simulink model "SVM_test2"  (R2020a)
settings: Solver=VariableStepAuto  StartTime=0.0  StopTime=Inf  FixedStep=Ts/2  RelTol=1e-3
PostLoadFcn:
  | , if any(exist('dsrtsu_mdlpostloadfcn', 'file') ~= 0), dsrtsu_mdlpostloadfcn('Execute', bdroot); end,
InitFcn:
  | , if any(exist('rtifpga_mdlclblib', 'file') ~= 0), rtifpga_mdlclblib('Init', bdroot); end,
model workspace (MAT data in the model file):
  FPGA_SVM_test2_1_Register_1_1_1_write : Simulink.Signal (value not decoded)
  FPGA_SVM_test2_1_Register_2_1_1_write : Simulink.Signal (value not decoded)
  FPGA_SVM_test2_1_Register_3_1_1_write : Simulink.Signal (value not decoded)
  FPGA_SVM_test2_1_Register_4_1_1_write : Simulink.Signal (value not decoded)
  FPGA_SVM_test2_1_Register_5_1_1_write : Simulink.Signal (value not decoded)
  FPGA_SVM_test2_1_Register_6_1_1_write : Simulink.Signal (value not decoded)
  FPGA_SVM_test2_1_Register_7_1_1_write : Simulink.Signal (value not decoded)
values from neighbouring files (symbols this model uses):
  clamp_threshold = 400    [param.m]
  i_fixed_gain = 10*1000/(3*100)    (= 33.3333333333)    [param.m]
  ioa_gain = 1    [param.m]
  ioa_offset = 0.09    [param.m]
  iob_gain = 1    [param.m]
  iob_offset = 0.06    [param.m]
  isa_gain = 1    [param.m]
  isa_offset = 0.1    [param.m]
  isb_gain = 1    [param.m]
  isb_offset = 0.3    [param.m]
  N = 1000    [param.m]
  vca_gain = 1    [param.m]
  vca_offset = 0.8    [param.m]
  vcb_gain = 1    [param.m]
  vcb_offset = 1.7    [param.m]
  vcc_gain = 1    [param.m]
  vcc_offset = 3    [param.m]
  vclamp_gain = 10*(76000+47000)/(3*100*2.5)    (= 1640)    [param.m]
  vclamp_offset = 11.7    [param.m]
  vi_fixed_gain = 10*33000/(3*100*2.5)    (= 440)    [param.m]
  via_gain = 1    [param.m]
  via_offset = 1    [param.m]
  vib_gain = 1    [param.m]
  vib_offset = 0.8    [param.m]
  vic_gain = 1    [param.m]
  vic_offset = -0.35    [param.m]
  voa_fixed_gain = 10*30000/(3*100*2.5)    (= 400)    [param.m]
  voa_gain = 1    [param.m]
  voa_offset = 0.7    [param.m]
libraries: xbsIndex_r4 x466, rti1202lib_adc_class1 x12, rtiproclib x10, simulink x3, rtifpgainterfacelib x1, powerlib_meascontrol x1
(part 8 of 9)

== system SVM_test2/Subsystem/FPGA_XDATA_READ_BL4 ==
  CEP1 : xbsIndex_r4/Clock Enable Probe  inherit_constraints=off  block_type=ceprobe
      settings: infoedit="Clock enable extractor.  Produces a Boolean output that mirrors the hardware clock enable associated with the input sample rate.<br><br>Hardware notes: in hardware this block costs nothing."
  CEP3 : xbsIndex_r4/Clock Enable Probe  inherit_constraints=off  block_type=ceprobe
      settings: infoedit="Clock enable extractor.  Produces a Boolean output that mirrors the hardware clock enable associated with the input sample rate.<br><br>Hardware notes: in hardware this block costs nothing."
  Constant1 : xbsIndex_r4/Constant  const=1  gui_display_data_type=Fixed-point  arith_type=Boolean  n_bits=16  bin_pt=14  preci_type=Single  exp_width=8  frac_width=24  explicit_period=on  period=1*1e-08  equ=P=C  opselect=C  inp2=PCIN>>17  opr=+  inp1=P  carry=CIN  dbl_ovrd=off  block_type=constant
  Constant3 : xbsIndex_r4/Constant  const=1  gui_display_data_type=Fixed-point  arith_type=Boolean  n_bits=16  bin_pt=14  preci_type=Single  exp_width=8  frac_width=24  explicit_period=on  period=1*1e-08  equ=P=C  opselect=C  inp2=PCIN>>17  opr=+  inp1=P  carry=CIN  dbl_ovrd=off  block_type=constant
  Delay1 : xbsIndex_r4/Delay  rst=off  infoeditControl=Selection of Reset will increase slice count due to use of real FFs and instead of SRLs  en=off  latency=0  reg_retiming=off  dbl_ovrd=off  block_type=delay
  Delay3 : xbsIndex_r4/Delay  rst=off  infoeditControl=Selection of Reset will increase slice count due to use of real FFs and instead of SRLs  en=off  latency=0  reg_retiming=off  dbl_ovrd=off  block_type=delay
  Register1 : xbsIndex_r4/Register  init=0  rst=off  en=on  dbl_ovrd=off  block_type=register
  Register3 : xbsIndex_r4/Register  init=0  rst=off  en=on  dbl_ovrd=off  block_type=register
  phs_read_register : Subsystem
      mask init: same as SVM_test2/Subsystem/FPGA_XDATA_READ_BL1/phs_read_register
  xreg_003_dout : xbsIndex_r4/Gateway In  gui_display_data_type=Fixed-point  arith_type=Unsigned  n_bits=32  bin_pt=0  preci_type=Single  exp_width=8  frac_width=24  rows=1  columns=1  quantization="Round  (unbiased: +/- Inf)"  overflow=Saturate  period=1e-08  UseAsADC=off  ADCChannel='1'  interface=None  automatic_assignment=on  address_offset=hex2dec('00')  intf_name=''  intf_description=''  default_value=0  timing_constraint=None  locs_specified=off  LOCs={}  io_standard={}  inherit_from_input=off  hdl_port=on  dbl_ovrd=off  block_type=gatewayin
  xreg_003_dout_wr : xbsIndex_r4/Gateway In  gui_display_data_type=Fixed-point  arith_type=Unsigned  n_bits=1  bin_pt=0  preci_type=Single  exp_width=8  frac_width=24  rows=1  columns=1  quantization="Round  (unbiased: +/- Inf)"  overflow=Saturate  period=1e-08  UseAsADC=off  ADCChannel='1'  interface=None  automatic_assignment=on  address_offset=hex2dec('00')  intf_name=''  intf_description=''  default_value=0  timing_constraint=None  locs_specified=off  LOCs={}  io_standard={}  inherit_from_input=off  hdl_port=on  dbl_ovrd=off  block_type=gatewayin
  Data : Outport
  Data New : Outport  Port=2
  wires:
  [FPGA_SVM_test2_rtiFPGAtmp_1_Register_4_1_1_write] -> phs_read_register/1(data_i)
  phs_read_register/2(data_new_o) -> xreg_003_dout_wr/1
  phs_read_register/1(data_o) -> xreg_003_dout/1
  xreg_003_dout_wr/1 -> Register3/1
  CEP3/1 -> Register3/2
  Constant3/1 -> CEP3/1
  Delay3/1 -> Data New/1
  Register3/1 -> Delay3/1
  xreg_003_dout/1 -> Register1/1
  CEP1/1 -> Register1/2
  Constant1/1 -> CEP1/1
  Delay1/1 -> Data/1
  Register1/1 -> Delay1/1

== system SVM_test2/Subsystem/FPGA_XDATA_READ_BL5 ==
  CEP1 : xbsIndex_r4/Clock Enable Probe  inherit_constraints=off  block_type=ceprobe
      settings: infoedit="Clock enable extractor.  Produces a Boolean output that mirrors the hardware clock enable associated with the input sample rate.<br><br>Hardware notes: in hardware this block costs nothing."
  CEP3 : xbsIndex_r4/Clock Enable Probe  inherit_constraints=off  block_type=ceprobe
      settings: infoedit="Clock enable extractor.  Produces a Boolean output that mirrors the hardware clock enable associated with the input sample rate.<br><br>Hardware notes: in hardware this block costs nothing."
  Constant1 : xbsIndex_r4/Constant  const=1  gui_display_data_type=Fixed-point  arith_type=Boolean  n_bits=16  bin_pt=14  preci_type=Single  exp_width=8  frac_width=24  explicit_period=on  period=1*1e-08  equ=P=C  opselect=C  inp2=PCIN>>17  opr=+  inp1=P  carry=CIN  dbl_ovrd=off  block_type=constant
  Constant3 : xbsIndex_r4/Constant  const=1  gui_display_data_type=Fixed-point  arith_type=Boolean  n_bits=16  bin_pt=14  preci_type=Single  exp_width=8  frac_width=24  explicit_period=on  period=1*1e-08  equ=P=C  opselect=C  inp2=PCIN>>17  opr=+  inp1=P  carry=CIN  dbl_ovrd=off  block_type=constant
  Delay1 : xbsIndex_r4/Delay  rst=off  infoeditControl=Selection of Reset will increase slice count due to use of real FFs and instead of SRLs  en=off  latency=0  reg_retiming=off  dbl_ovrd=off  block_type=delay
  Delay3 : xbsIndex_r4/Delay  rst=off  infoeditControl=Selection of Reset will increase slice count due to use of real FFs and instead of SRLs  en=off  latency=0  reg_retiming=off  dbl_ovrd=off  block_type=delay
  Register1 : xbsIndex_r4/Register  init=0  rst=off  en=on  dbl_ovrd=off  block_type=register
  Register3 : xbsIndex_r4/Register  init=0  rst=off  en=on  dbl_ovrd=off  block_type=register
  phs_read_register : Subsystem
      mask init: same as SVM_test2/Subsystem/FPGA_XDATA_READ_BL1/phs_read_register
  xreg_004_dout : xbsIndex_r4/Gateway In  gui_display_data_type=Fixed-point  arith_type=Unsigned  n_bits=32  bin_pt=0  preci_type=Single  exp_width=8  frac_width=24  rows=1  columns=1  quantization="Round  (unbiased: +/- Inf)"  overflow=Saturate  period=1e-08  UseAsADC=off  ADCChannel='1'  interface=None  automatic_assignment=on  address_offset=hex2dec('00')  intf_name=''  intf_description=''  default_value=0  timing_constraint=None  locs_specified=off  LOCs={}  io_standard={}  inherit_from_input=off  hdl_port=on  dbl_ovrd=off  block_type=gatewayin
  xreg_004_dout_wr : xbsIndex_r4/Gateway In  gui_display_data_type=Fixed-point  arith_type=Unsigned  n_bits=1  bin_pt=0  preci_type=Single  exp_width=8  frac_width=24  rows=1  columns=1  quantization="Round  (unbiased: +/- Inf)"  overflow=Saturate  period=1e-08  UseAsADC=off  ADCChannel='1'  interface=None  automatic_assignment=on  address_offset=hex2dec('00')  intf_name=''  intf_description=''  default_value=0  timing_constraint=None  locs_specified=off  LOCs={}  io_standard={}  inherit_from_input=off  hdl_port=on  dbl_ovrd=off  block_type=gatewayin
  Data : Outport
  Data New : Outport  Port=2
  wires:
  [FPGA_SVM_test2_rtiFPGAtmp_1_Register_5_1_1_write] -> phs_read_register/1(data_i)
  phs_read_register/2(data_new_o) -> xreg_004_dout_wr/1
  phs_read_register/1(data_o) -> xreg_004_dout/1
  xreg_004_dout_wr/1 -> Register3/1
  CEP3/1 -> Register3/2
  Constant3/1 -> CEP3/1
  Delay3/1 -> Data New/1
  Register3/1 -> Delay3/1
  xreg_004_dout/1 -> Register1/1
  CEP1/1 -> Register1/2
  Constant1/1 -> CEP1/1
  Delay1/1 -> Data/1
  Register1/1 -> Delay1/1

== system SVM_test2/Subsystem/FPGA_XDATA_READ_BL6 ==
  CEP1 : xbsIndex_r4/Clock Enable Probe  inherit_constraints=off  block_type=ceprobe
      settings: infoedit="Clock enable extractor.  Produces a Boolean output that mirrors the hardware clock enable associated with the input sample rate.<br><br>Hardware notes: in hardware this block costs nothing."
  CEP3 : xbsIndex_r4/Clock Enable Probe  inherit_constraints=off  block_type=ceprobe
      settings: infoedit="Clock enable extractor.  Produces a Boolean output that mirrors the hardware clock enable associated with the input sample rate.<br><br>Hardware notes: in hardware this block costs nothing."
  Constant1 : xbsIndex_r4/Constant  const=1  gui_display_data_type=Fixed-point  arith_type=Boolean  n_bits=16  bin_pt=14  preci_type=Single  exp_width=8  frac_width=24  explicit_period=on  period=1*1e-08  equ=P=C  opselect=C  inp2=PCIN>>17  opr=+  inp1=P  carry=CIN  dbl_ovrd=off  block_type=constant
  Constant3 : xbsIndex_r4/Constant  const=1  gui_display_data_type=Fixed-point  arith_type=Boolean  n_bits=16  bin_pt=14  preci_type=Single  exp_width=8  frac_width=24  explicit_period=on  period=1*1e-08  equ=P=C  opselect=C  inp2=PCIN>>17  opr=+  inp1=P  carry=CIN  dbl_ovrd=off  block_type=constant
  Delay1 : xbsIndex_r4/Delay  rst=off  infoeditControl=Selection of Reset will increase slice count due to use of real FFs and instead of SRLs  en=off  latency=0  reg_retiming=off  dbl_ovrd=off  block_type=delay
  Delay3 : xbsIndex_r4/Delay  rst=off  infoeditControl=Selection of Reset will increase slice count due to use of real FFs and instead of SRLs  en=off  latency=0  reg_retiming=off  dbl_ovrd=off  block_type=delay
  Register1 : xbsIndex_r4/Register  init=0  rst=off  en=on  dbl_ovrd=off  block_type=register
  Register3 : xbsIndex_r4/Register  init=0  rst=off  en=on  dbl_ovrd=off  block_type=register
  phs_read_register : Subsystem
      mask init: same as SVM_test2/Subsystem/FPGA_XDATA_READ_BL1/phs_read_register
  xreg_005_dout : xbsIndex_r4/Gateway In  gui_display_data_type=Fixed-point  arith_type=Unsigned  n_bits=32  bin_pt=0  preci_type=Single  exp_width=8  frac_width=24  rows=1  columns=1  quantization="Round  (unbiased: +/- Inf)"  overflow=Saturate  period=1e-08  UseAsADC=off  ADCChannel='1'  interface=None  automatic_assignment=on  address_offset=hex2dec('00')  intf_name=''  intf_description=''  default_value=0  timing_constraint=None  locs_specified=off  LOCs={}  io_standard={}  inherit_from_input=off  hdl_port=on  dbl_ovrd=off  block_type=gatewayin
  xreg_005_dout_wr : xbsIndex_r4/Gateway In  gui_display_data_type=Fixed-point  arith_type=Unsigned  n_bits=1  bin_pt=0  preci_type=Single  exp_width=8  frac_width=24  rows=1  columns=1  quantization="Round  (unbiased: +/- Inf)"  overflow=Saturate  period=1e-08  UseAsADC=off  ADCChannel='1'  interface=None  automatic_assignment=on  address_offset=hex2dec('00')  intf_name=''  intf_description=''  default_value=0  timing_constraint=None  locs_specified=off  LOCs={}  io_standard={}  inherit_from_input=off  hdl_port=on  dbl_ovrd=off  block_type=gatewayin
  Data : Outport
  Data New : Outport  Port=2
  wires:
  [FPGA_SVM_test2_rtiFPGAtmp_1_Register_6_1_1_write] -> phs_read_register/1(data_i)
  phs_read_register/2(data_new_o) -> xreg_005_dout_wr/1
  phs_read_register/1(data_o) -> xreg_005_dout/1
  xreg_005_dout_wr/1 -> Register3/1
  CEP3/1 -> Register3/2
  Constant3/1 -> CEP3/1
  Delay3/1 -> Data New/1
  Register3/1 -> Delay3/1
  xreg_005_dout/1 -> Register1/1
  CEP1/1 -> Register1/2
  Constant1/1 -> CEP1/1
  Delay1/1 -> Data/1
  Register1/1 -> Delay1/1

== system SVM_test2/Subsystem/FPGA_XDATA_READ_BL7 ==
  CEP1 : xbsIndex_r4/Clock Enable Probe  inherit_constraints=off  block_type=ceprobe
      settings: infoedit="Clock enable extractor.  Produces a Boolean output that mirrors the hardware clock enable associated with the input sample rate.<br><br>Hardware notes: in hardware this block costs nothing."
  CEP3 : xbsIndex_r4/Clock Enable Probe  inherit_constraints=off  block_type=ceprobe
      settings: infoedit="Clock enable extractor.  Produces a Boolean output that mirrors the hardware clock enable associated with the input sample rate.<br><br>Hardware notes: in hardware this block costs nothing."
  Constant1 : xbsIndex_r4/Constant  const=1  gui_display_data_type=Fixed-point  arith_type=Boolean  n_bits=16  bin_pt=14  preci_type=Single  exp_width=8  frac_width=24  explicit_period=on  period=1*1e-08  equ=P=C  opselect=C  inp2=PCIN>>17  opr=+  inp1=P  carry=CIN  dbl_ovrd=off  block_type=constant
  Constant3 : xbsIndex_r4/Constant  const=1  gui_display_data_type=Fixed-point  arith_type=Boolean  n_bits=16  bin_pt=14  preci_type=Single  exp_width=8  frac_width=24  explicit_period=on  period=1*1e-08  equ=P=C  opselect=C  inp2=PCIN>>17  opr=+  inp1=P  carry=CIN  dbl_ovrd=off  block_type=constant
  Delay1 : xbsIndex_r4/Delay  rst=off  infoeditControl=Selection of Reset will increase slice count due to use of real FFs and instead of SRLs  en=off  latency=0  reg_retiming=off  dbl_ovrd=off  block_type=delay
  Delay3 : xbsIndex_r4/Delay  rst=off  infoeditControl=Selection of Reset will increase slice count due to use of real FFs and instead of SRLs  en=off  latency=0  reg_retiming=off  dbl_ovrd=off  block_type=delay
  Register1 : xbsIndex_r4/Register  init=0  rst=off  en=on  dbl_ovrd=off  block_type=register
  Register3 : xbsIndex_r4/Register  init=0  rst=off  en=on  dbl_ovrd=off  block_type=register
  phs_read_register : Subsystem
      mask init: same as SVM_test2/Subsystem/FPGA_XDATA_READ_BL1/phs_read_register
  xreg_006_dout : xbsIndex_r4/Gateway In  gui_display_data_type=Fixed-point  arith_type=Unsigned  n_bits=32  bin_pt=0  preci_type=Single  exp_width=8  frac_width=24  rows=1  columns=1  quantization="Round  (unbiased: +/- Inf)"  overflow=Saturate  period=1e-08  UseAsADC=off  ADCChannel='1'  interface=None  automatic_assignment=on  address_offset=hex2dec('00')  intf_name=''  intf_description=''  default_value=0  timing_constraint=None  locs_specified=off  LOCs={}  io_standard={}  inherit_from_input=off  hdl_port=on  dbl_ovrd=off  block_type=gatewayin
  xreg_006_dout_wr : xbsIndex_r4/Gateway In  gui_display_data_type=Fixed-point  arith_type=Unsigned  n_bits=1  bin_pt=0  preci_type=Single  exp_width=8  frac_width=24  rows=1  columns=1  quantization="Round  (unbiased: +/- Inf)"  overflow=Saturate  period=1e-08  UseAsADC=off  ADCChannel='1'  interface=None  automatic_assignment=on  address_offset=hex2dec('00')  intf_name=''  intf_description=''  default_value=0  timing_constraint=None  locs_specified=off  LOCs={}  io_standard={}  inherit_from_input=off  hdl_port=on  dbl_ovrd=off  block_type=gatewayin
  Data : Outport
  Data New : Outport  Port=2
  wires:
  [FPGA_SVM_test2_rtiFPGAtmp_1_Register_7_1_1_write] -> phs_read_register/1(data_i)
  phs_read_register/2(data_new_o) -> xreg_006_dout_wr/1
  phs_read_register/1(data_o) -> xreg_006_dout/1
  xreg_006_dout_wr/1 -> Register3/1
  CEP3/1 -> Register3/2
  Constant3/1 -> CEP3/1
  Delay3/1 -> Data New/1
  Register3/1 -> Delay3/1
  xreg_006_dout/1 -> Register1/1
  CEP1/1 -> Register1/2
  Constant1/1 -> CEP1/1
  Delay1/1 -> Data/1
  Register1/1 -> Delay1/1

== system SVM_test2/RTI Data/RTI Data Store/RTI Data Store ==
  RTI Data Store : Subsystem  mask(RTI_DATA_STORE){}
      mask help:
      | RTI Data Store Block. This block is used by RTI to store internal model dependent data. Deleting this block will result in data loss.
      |
      | NEVER DELETE, COPY, OR MODIFY THIS BLOCK!
      mask Help:
      | RTI Data Store Block. This block is used by RTI to store internal model dependent data. Deleting this block will result in data loss.
      | 
      | NEVER DELETE, COPY, OR MODIFY THIS BLOCK!
      mask Display: text(0.5, 0.5, ' ', 'HorizontalAlignment', 'center');

== system SVM_test2/Subsystem/FPGA_INT_BL1/phs_interrupt ==
  note: Subsystem simulating the communication
      | function specific behaviour. This is how the
      | FPGA framework driver takes effect on the data.
  note: Subsystem simulating the phs bus
      | access via RTLib functions.
  data_i : Inport
  com_fct_model : Subsystem
  phs/rtlib_sim_model : Subsystem
  data_o : Outport  VectorParamsAs1DForOutWhenUnconnected=off
  wires:
  data_i/1 -> com_fct_model/1(data_i1)
  com_fct_model/1(data_o1) -> phs/rtlib_sim_model/1(data_i1)
  phs/rtlib_sim_model/1(data_o1) -> data_o/1

== system SVM_test2/Subsystem/FPGA_INT_BL2/phs_interrupt ==
  note: Subsystem simulating the communication
      | function specific behaviour. This is how the
      | FPGA framework driver takes effect on the data.
  note: Subsystem simulating the phs bus
      | access via RTLib functions.
  data_i : Inport
  com_fct_model : Subsystem
  phs/rtlib_sim_model : Subsystem
  data_o : Outport  VectorParamsAs1DForOutWhenUnconnected=off
  wires:
  data_i/1 -> com_fct_model/1(data_i1)
  com_fct_model/1(data_o1) -> phs/rtlib_sim_model/1(data_i1)
  phs/rtlib_sim_model/1(data_o1) -> data_o/1

== system SVM_test2/Subsystem/FPGA_IO_WRITE_BL1/dig_inout_tp1 ==
  note: The Digital In value is simulated by Threshold voltage detection.
  note: The nominal input range is NOT simulated because
      | the HW does not saturate according to the input range.
  data_in_i : Inport
  enable_i : Inport  Port=2
  data_out_i : Inport  Port=3
  direction_i : Inport  Port=4
  Data Type Conversion : DataTypeConversion
  Data Type Conversion1 : DataTypeConversion
  Disabled Input Value : Constant  Value=0
  Disabled Output Value : Constant  Value=0
  Invert : Constant  Value=inverted_dio
  Invert1 : Constant  Value=inverted_dio
  Inverter : Logic  Operator=NOT  AllPortsSameDT=off  OutDataTypeStr=boolean
  Inverter1 : Logic  AllPortsSameDT=off  OutDataTypeStr=boolean
  Inverter2 : Logic  Operator=NOT  AllPortsSameDT=off  OutDataTypeStr=boolean
  Inverter3 : Logic  AllPortsSameDT=off  OutDataTypeStr=boolean
  Inverter4 : Logic  Operator=NOT  AllPortsSameDT=off  OutDataTypeStr=boolean
  Relational Operator : RelationalOperator  OutDataTypeStr=boolean  RndMeth=Nearest
  Switch{,1..3} (4 alike) : Switch  Threshold=1
  Threshold Voltage : Constant  Value=2
  Voltage : Gain  Gain=voltage  ParamDataTypeStr=float('double')
  data_in_o : Outport  VectorParamsAs1DForOutWhenUnconnected=off
  data_out_o : Outport  Port=2  VectorParamsAs1DForOutWhenUnconnected=off
  wires:
  data_in_i/1 -> Relational Operator/1
  Threshold Voltage/1 -> Relational Operator/2
  Disabled Input Value/1 -> Switch/3
  Switch1/1 -> data_in_o/1
  Invert/1 -> Switch1/2
  Inverter/1 -> Switch1/1
  Relational Operator/1 -> Switch/1
  Switch/1 -> Inverter/1, Switch1/3
  enable_i/1 -> Data Type Conversion/1
  Inverter1/1 -> Switch/2
  direction_i/1 -> Data Type Conversion1/1
  Inverter2/1 -> Inverter1/2
  Disabled Output Value/1 -> Switch2/3
  Inverter3/1 -> Switch2/2
  data_out_i/1 -> Switch2/1
  Invert1/1 -> Switch3/2
  Inverter4/1 -> Switch3/1
  Switch2/1 -> Inverter4/1, Switch3/3
  Switch3/1 -> Voltage/1
  Data Type Conversion/1 -> Inverter1/1, Inverter3/1
  Data Type Conversion1/1 -> Inverter2/1, Inverter3/2
  Voltage/1 -> data_out_o/1

== system SVM_test2/Subsystem/FPGA_IO_WRITE_BL10/dig_inout_tp1 ==
  note: The Digital In value is simulated by Threshold voltage detection.
  note: The nominal input range is NOT simulated because
      | the HW does not saturate according to the input range.
  data_in_i : Inport
  enable_i : Inport  Port=2
  data_out_i : Inport  Port=3
  direction_i : Inport  Port=4
  Data Type Conversion : DataTypeConversion
  Data Type Conversion1 : DataTypeConversion
  Disabled Input Value : Constant  Value=0
  Disabled Output Value : Constant  Value=0
  Invert : Constant  Value=inverted_dio
  Invert1 : Constant  Value=inverted_dio
  Inverter : Logic  Operator=NOT  AllPortsSameDT=off  OutDataTypeStr=boolean
  Inverter1 : Logic  AllPortsSameDT=off  OutDataTypeStr=boolean
  Inverter2 : Logic  Operator=NOT  AllPortsSameDT=off  OutDataTypeStr=boolean
  Inverter3 : Logic  AllPortsSameDT=off  OutDataTypeStr=boolean
  Inverter4 : Logic  Operator=NOT  AllPortsSameDT=off  OutDataTypeStr=boolean
  Relational Operator : RelationalOperator  OutDataTypeStr=boolean  RndMeth=Nearest
  Switch{,1..3} (4 alike) : Switch  Threshold=1
  Threshold Voltage : Constant  Value=2
  Voltage : Gain  Gain=voltage  ParamDataTypeStr=float('double')
  data_in_o : Outport  VectorParamsAs1DForOutWhenUnconnected=off
  data_out_o : Outport  Port=2  VectorParamsAs1DForOutWhenUnconnected=off
  wires:
  data_in_i/1 -> Relational Operator/1
  Threshold Voltage/1 -> Relational Operator/2
  Disabled Input Value/1 -> Switch/3
  Switch1/1 -> data_in_o/1
  Invert/1 -> Switch1/2
  Inverter/1 -> Switch1/1
  Relational Operator/1 -> Switch/1
  Switch/1 -> Inverter/1, Switch1/3
  enable_i/1 -> Data Type Conversion/1
  Inverter1/1 -> Switch/2
  direction_i/1 -> Data Type Conversion1/1
  Inverter2/1 -> Inverter1/2
  Disabled Output Value/1 -> Switch2/3
  Inverter3/1 -> Switch2/2
  data_out_i/1 -> Switch2/1
  Invert1/1 -> Switch3/2
  Inverter4/1 -> Switch3/1
  Switch2/1 -> Inverter4/1, Switch3/3
  Switch3/1 -> Voltage/1
  Data Type Conversion/1 -> Inverter1/1, Inverter3/1
  Data Type Conversion1/1 -> Inverter2/1, Inverter3/2
  Voltage/1 -> data_out_o/1

== system SVM_test2/Subsystem/FPGA_IO_WRITE_BL11/dig_inout_tp1 ==
  note: The Digital In value is simulated by Threshold voltage detection.
  note: The nominal input range is NOT simulated because
      | the HW does not saturate according to the input range.
  data_in_i : Inport
  enable_i : Inport  Port=2
  data_out_i : Inport  Port=3
  direction_i : Inport  Port=4
  Data Type Conversion : DataTypeConversion
  Data Type Conversion1 : DataTypeConversion
  Disabled Input Value : Constant  Value=0
  Disabled Output Value : Constant  Value=0
  Invert : Constant  Value=inverted_dio
  Invert1 : Constant  Value=inverted_dio
  Inverter : Logic  Operator=NOT  AllPortsSameDT=off  OutDataTypeStr=boolean
  Inverter1 : Logic  AllPortsSameDT=off  OutDataTypeStr=boolean
  Inverter2 : Logic  Operator=NOT  AllPortsSameDT=off  OutDataTypeStr=boolean
  Inverter3 : Logic  AllPortsSameDT=off  OutDataTypeStr=boolean
  Inverter4 : Logic  Operator=NOT  AllPortsSameDT=off  OutDataTypeStr=boolean
  Relational Operator : RelationalOperator  OutDataTypeStr=boolean  RndMeth=Nearest
  Switch{,1..3} (4 alike) : Switch  Threshold=1
  Threshold Voltage : Constant  Value=2
  Voltage : Gain  Gain=voltage  ParamDataTypeStr=float('double')
  data_in_o : Outport  VectorParamsAs1DForOutWhenUnconnected=off
  data_out_o : Outport  Port=2  VectorParamsAs1DForOutWhenUnconnected=off
  wires:
  data_in_i/1 -> Relational Operator/1
  Threshold Voltage/1 -> Relational Operator/2
  Disabled Input Value/1 -> Switch/3
  Switch1/1 -> data_in_o/1
  Invert/1 -> Switch1/2
  Inverter/1 -> Switch1/1
  Relational Operator/1 -> Switch/1
  Switch/1 -> Inverter/1, Switch1/3
  enable_i/1 -> Data Type Conversion/1
  Inverter1/1 -> Switch/2
  direction_i/1 -> Data Type Conversion1/1
  Inverter2/1 -> Inverter1/2
  Disabled Output Value/1 -> Switch2/3
  Inverter3/1 -> Switch2/2
  data_out_i/1 -> Switch2/1
  Invert1/1 -> Switch3/2
  Inverter4/1 -> Switch3/1
  Switch2/1 -> Inverter4/1, Switch3/3
  Switch3/1 -> Voltage/1
  Data Type Conversion/1 -> Inverter1/1, Inverter3/1
  Data Type Conversion1/1 -> Inverter2/1, Inverter3/2
  Voltage/1 -> data_out_o/1

== system SVM_test2/Subsystem/FPGA_IO_WRITE_BL12/dig_inout_tp1 ==
  note: The Digital In value is simulated by Threshold voltage detection.
  note: The nominal input range is NOT simulated because
      | the HW does not saturate according to the input range.
  data_in_i : Inport
  enable_i : Inport  Port=2
  data_out_i : Inport  Port=3
  direction_i : Inport  Port=4
  Data Type Conversion : DataTypeConversion
  Data Type Conversion1 : DataTypeConversion
  Disabled Input Value : Constant  Value=0
  Disabled Output Value : Constant  Value=0
  Invert : Constant  Value=inverted_dio
  Invert1 : Constant  Value=inverted_dio
  Inverter : Logic  Operator=NOT  AllPortsSameDT=off  OutDataTypeStr=boolean
  Inverter1 : Logic  AllPortsSameDT=off  OutDataTypeStr=boolean
  Inverter2 : Logic  Operator=NOT  AllPortsSameDT=off  OutDataTypeStr=boolean
  Inverter3 : Logic  AllPortsSameDT=off  OutDataTypeStr=boolean
  Inverter4 : Logic  Operator=NOT  AllPortsSameDT=off  OutDataTypeStr=boolean
  Relational Operator : RelationalOperator  OutDataTypeStr=boolean  RndMeth=Nearest
  Switch{,1..3} (4 alike) : Switch  Threshold=1
  Threshold Voltage : Constant  Value=2
  Voltage : Gain  Gain=voltage  ParamDataTypeStr=float('double')
  data_in_o : Outport  VectorParamsAs1DForOutWhenUnconnected=off
  data_out_o : Outport  Port=2  VectorParamsAs1DForOutWhenUnconnected=off
  wires:
  data_in_i/1 -> Relational Operator/1
  Threshold Voltage/1 -> Relational Operator/2
  Disabled Input Value/1 -> Switch/3
  Switch1/1 -> data_in_o/1
  Invert/1 -> Switch1/2
  Inverter/1 -> Switch1/1
  Relational Operator/1 -> Switch/1
  Switch/1 -> Inverter/1, Switch1/3
  enable_i/1 -> Data Type Conversion/1
  Inverter1/1 -> Switch/2
  direction_i/1 -> Data Type Conversion1/1
  Inverter2/1 -> Inverter1/2
  Disabled Output Value/1 -> Switch2/3
  Inverter3/1 -> Switch2/2
  data_out_i/1 -> Switch2/1
  Invert1/1 -> Switch3/2
  Inverter4/1 -> Switch3/1
  Switch2/1 -> Inverter4/1, Switch3/3
  Switch3/1 -> Voltage/1
  Data Type Conversion/1 -> Inverter1/1, Inverter3/1
  Data Type Conversion1/1 -> Inverter2/1, Inverter3/2
  Voltage/1 -> data_out_o/1

== system SVM_test2/Subsystem/FPGA_IO_WRITE_BL13/dig_inout_tp1 ==
  note: The Digital In value is simulated by Threshold voltage detection.
  note: The nominal input range is NOT simulated because
      | the HW does not saturate according to the input range.
  data_in_i : Inport
  enable_i : Inport  Port=2
  data_out_i : Inport  Port=3
  direction_i : Inport  Port=4
  Data Type Conversion : DataTypeConversion
  Data Type Conversion1 : DataTypeConversion
  Disabled Input Value : Constant  Value=0
  Disabled Output Value : Constant  Value=0
  Invert : Constant  Value=inverted_dio
  Invert1 : Constant  Value=inverted_dio
  Inverter : Logic  Operator=NOT  AllPortsSameDT=off  OutDataTypeStr=boolean
  Inverter1 : Logic  AllPortsSameDT=off  OutDataTypeStr=boolean
  Inverter2 : Logic  Operator=NOT  AllPortsSameDT=off  OutDataTypeStr=boolean
  Inverter3 : Logic  AllPortsSameDT=off  OutDataTypeStr=boolean
  Inverter4 : Logic  Operator=NOT  AllPortsSameDT=off  OutDataTypeStr=boolean
  Relational Operator : RelationalOperator  OutDataTypeStr=boolean  RndMeth=Nearest
  Switch{,1..3} (4 alike) : Switch  Threshold=1
  Threshold Voltage : Constant  Value=2
  Voltage : Gain  Gain=voltage  ParamDataTypeStr=float('double')
  data_in_o : Outport  VectorParamsAs1DForOutWhenUnconnected=off
  data_out_o : Outport  Port=2  VectorParamsAs1DForOutWhenUnconnected=off
  wires:
  data_in_i/1 -> Relational Operator/1
  Threshold Voltage/1 -> Relational Operator/2
  Disabled Input Value/1 -> Switch/3
  Switch1/1 -> data_in_o/1
  Invert/1 -> Switch1/2
  Inverter/1 -> Switch1/1
  Relational Operator/1 -> Switch/1
  Switch/1 -> Inverter/1, Switch1/3
  enable_i/1 -> Data Type Conversion/1
  Inverter1/1 -> Switch/2
  direction_i/1 -> Data Type Conversion1/1
  Inverter2/1 -> Inverter1/2
  Disabled Output Value/1 -> Switch2/3
  Inverter3/1 -> Switch2/2
  data_out_i/1 -> Switch2/1
  Invert1/1 -> Switch3/2
  Inverter4/1 -> Switch3/1
  Switch2/1 -> Inverter4/1, Switch3/3
  Switch3/1 -> Voltage/1
  Data Type Conversion/1 -> Inverter1/1, Inverter3/1
  Data Type Conversion1/1 -> Inverter2/1, Inverter3/2
  Voltage/1 -> data_out_o/1

== system SVM_test2/Subsystem/FPGA_IO_WRITE_BL14/dig_inout_tp1 ==
  note: The Digital In value is simulated by Threshold voltage detection.
  note: The nominal input range is NOT simulated because
      | the HW does not saturate according to the input range.
  data_in_i : Inport
  enable_i : Inport  Port=2
  data_out_i : Inport  Port=3
  direction_i : Inport  Port=4
  Data Type Conversion : DataTypeConversion
  Data Type Conversion1 : DataTypeConversion
  Disabled Input Value : Constant  Value=0
  Disabled Output Value : Constant  Value=0
  Invert : Constant  Value=inverted_dio
  Invert1 : Constant  Value=inverted_dio
  Inverter : Logic  Operator=NOT  AllPortsSameDT=off  OutDataTypeStr=boolean
  Inverter1 : Logic  AllPortsSameDT=off  OutDataTypeStr=boolean
  Inverter2 : Logic  Operator=NOT  AllPortsSameDT=off  OutDataTypeStr=boolean
  Inverter3 : Logic  AllPortsSameDT=off  OutDataTypeStr=boolean
  Inverter4 : Logic  Operator=NOT  AllPortsSameDT=off  OutDataTypeStr=boolean
  Relational Operator : RelationalOperator  OutDataTypeStr=boolean  RndMeth=Nearest
  Switch{,1..3} (4 alike) : Switch  Threshold=1
  Threshold Voltage : Constant  Value=2
  Voltage : Gain  Gain=voltage  ParamDataTypeStr=float('double')
  data_in_o : Outport  VectorParamsAs1DForOutWhenUnconnected=off
  data_out_o : Outport  Port=2  VectorParamsAs1DForOutWhenUnconnected=off
  wires:
  data_in_i/1 -> Relational Operator/1
  Threshold Voltage/1 -> Relational Operator/2
  Disabled Input Value/1 -> Switch/3
  Switch1/1 -> data_in_o/1
  Invert/1 -> Switch1/2
  Inverter/1 -> Switch1/1
  Relational Operator/1 -> Switch/1
  Switch/1 -> Inverter/1, Switch1/3
  enable_i/1 -> Data Type Conversion/1
  Inverter1/1 -> Switch/2
  direction_i/1 -> Data Type Conversion1/1
  Inverter2/1 -> Inverter1/2
  Disabled Output Value/1 -> Switch2/3
  Inverter3/1 -> Switch2/2
  data_out_i/1 -> Switch2/1
  Invert1/1 -> Switch3/2
  Inverter4/1 -> Switch3/1
  Switch2/1 -> Inverter4/1, Switch3/3
  Switch3/1 -> Voltage/1
  Data Type Conversion/1 -> Inverter1/1, Inverter3/1
  Data Type Conversion1/1 -> Inverter2/1, Inverter3/2
  Voltage/1 -> data_out_o/1

== system SVM_test2/Subsystem/FPGA_IO_WRITE_BL15/dig_inout_tp1 ==
  note: The Digital In value is simulated by Threshold voltage detection.
  note: The nominal input range is NOT simulated because
      | the HW does not saturate according to the input range.
  data_in_i : Inport
  enable_i : Inport  Port=2
  data_out_i : Inport  Port=3
  direction_i : Inport  Port=4
  Data Type Conversion : DataTypeConversion
  Data Type Conversion1 : DataTypeConversion
  Disabled Input Value : Constant  Value=0
  Disabled Output Value : Constant  Value=0
  Invert : Constant  Value=inverted_dio
  Invert1 : Constant  Value=inverted_dio
  Inverter : Logic  Operator=NOT  AllPortsSameDT=off  OutDataTypeStr=boolean
  Inverter1 : Logic  AllPortsSameDT=off  OutDataTypeStr=boolean
  Inverter2 : Logic  Operator=NOT  AllPortsSameDT=off  OutDataTypeStr=boolean
  Inverter3 : Logic  AllPortsSameDT=off  OutDataTypeStr=boolean
  Inverter4 : Logic  Operator=NOT  AllPortsSameDT=off  OutDataTypeStr=boolean
  Relational Operator : RelationalOperator  OutDataTypeStr=boolean  RndMeth=Nearest
  Switch{,1..3} (4 alike) : Switch  Threshold=1
  Threshold Voltage : Constant  Value=2
  Voltage : Gain  Gain=voltage  ParamDataTypeStr=float('double')
  data_in_o : Outport  VectorParamsAs1DForOutWhenUnconnected=off
  data_out_o : Outport  Port=2  VectorParamsAs1DForOutWhenUnconnected=off
  wires:
  data_in_i/1 -> Relational Operator/1
  Threshold Voltage/1 -> Relational Operator/2
  Disabled Input Value/1 -> Switch/3
  Switch1/1 -> data_in_o/1
  Invert/1 -> Switch1/2
  Inverter/1 -> Switch1/1
  Relational Operator/1 -> Switch/1
  Switch/1 -> Inverter/1, Switch1/3
  enable_i/1 -> Data Type Conversion/1
  Inverter1/1 -> Switch/2
  direction_i/1 -> Data Type Conversion1/1
  Inverter2/1 -> Inverter1/2
  Disabled Output Value/1 -> Switch2/3
  Inverter3/1 -> Switch2/2
  data_out_i/1 -> Switch2/1
  Invert1/1 -> Switch3/2
  Inverter4/1 -> Switch3/1
  Switch2/1 -> Inverter4/1, Switch3/3
  Switch3/1 -> Voltage/1
  Data Type Conversion/1 -> Inverter1/1, Inverter3/1
  Data Type Conversion1/1 -> Inverter2/1, Inverter3/2
  Voltage/1 -> data_out_o/1

== system SVM_test2/Subsystem/FPGA_IO_WRITE_BL16/dig_inout_tp1 ==
  note: The Digital In value is simulated by Threshold voltage detection.
  note: The nominal input range is NOT simulated because
      | the HW does not saturate according to the input range.
  data_in_i : Inport
  enable_i : Inport  Port=2
  data_out_i : Inport  Port=3
  direction_i : Inport  Port=4
  Data Type Conversion : DataTypeConversion
  Data Type Conversion1 : DataTypeConversion
  Disabled Input Value : Constant  Value=0
  Disabled Output Value : Constant  Value=0
  Invert : Constant  Value=inverted_dio
  Invert1 : Constant  Value=inverted_dio
  Inverter : Logic  Operator=NOT  AllPortsSameDT=off  OutDataTypeStr=boolean
  Inverter1 : Logic  AllPortsSameDT=off  OutDataTypeStr=boolean
  Inverter2 : Logic  Operator=NOT  AllPortsSameDT=off  OutDataTypeStr=boolean
  Inverter3 : Logic  AllPortsSameDT=off  OutDataTypeStr=boolean
  Inverter4 : Logic  Operator=NOT  AllPortsSameDT=off  OutDataTypeStr=boolean
  Relational Operator : RelationalOperator  OutDataTypeStr=boolean  RndMeth=Nearest
  Switch{,1..3} (4 alike) : Switch  Threshold=1
  Threshold Voltage : Constant  Value=2
  Voltage : Gain  Gain=voltage  ParamDataTypeStr=float('double')
  data_in_o : Outport  VectorParamsAs1DForOutWhenUnconnected=off
  data_out_o : Outport  Port=2  VectorParamsAs1DForOutWhenUnconnected=off
  wires:
  data_in_i/1 -> Relational Operator/1
  Threshold Voltage/1 -> Relational Operator/2
  Disabled Input Value/1 -> Switch/3
  Switch1/1 -> data_in_o/1
  Invert/1 -> Switch1/2
  Inverter/1 -> Switch1/1
  Relational Operator/1 -> Switch/1
  Switch/1 -> Inverter/1, Switch1/3
  enable_i/1 -> Data Type Conversion/1
  Inverter1/1 -> Switch/2
  direction_i/1 -> Data Type Conversion1/1
  Inverter2/1 -> Inverter1/2
  Disabled Output Value/1 -> Switch2/3
  Inverter3/1 -> Switch2/2
  data_out_i/1 -> Switch2/1
  Invert1/1 -> Switch3/2
  Inverter4/1 -> Switch3/1
  Switch2/1 -> Inverter4/1, Switch3/3
  Switch3/1 -> Voltage/1
  Data Type Conversion/1 -> Inverter1/1, Inverter3/1
  Data Type Conversion1/1 -> Inverter2/1, Inverter3/2
  Voltage/1 -> data_out_o/1

== system SVM_test2/Subsystem/FPGA_IO_WRITE_BL17/dig_inout_tp1 ==
  note: The Digital In value is simulated by Threshold voltage detection.
  note: The nominal input range is NOT simulated because
      | the HW does not saturate according to the input range.
  data_in_i : Inport
  enable_i : Inport  Port=2
  data_out_i : Inport  Port=3
  direction_i : Inport  Port=4
  Data Type Conversion : DataTypeConversion
  Data Type Conversion1 : DataTypeConversion
  Disabled Input Value : Constant  Value=0
  Disabled Output Value : Constant  Value=0
  Invert : Constant  Value=inverted_dio
  Invert1 : Constant  Value=inverted_dio
  Inverter : Logic  Operator=NOT  AllPortsSameDT=off  OutDataTypeStr=boolean
  Inverter1 : Logic  AllPortsSameDT=off  OutDataTypeStr=boolean
  Inverter2 : Logic  Operator=NOT  AllPortsSameDT=off  OutDataTypeStr=boolean
  Inverter3 : Logic  AllPortsSameDT=off  OutDataTypeStr=boolean
  Inverter4 : Logic  Operator=NOT  AllPortsSameDT=off  OutDataTypeStr=boolean
  Relational Operator : RelationalOperator  OutDataTypeStr=boolean  RndMeth=Nearest
  Switch{,1..3} (4 alike) : Switch  Threshold=1
  Threshold Voltage : Constant  Value=2
  Voltage : Gain  Gain=voltage  ParamDataTypeStr=float('double')
  data_in_o : Outport  VectorParamsAs1DForOutWhenUnconnected=off
  data_out_o : Outport  Port=2  VectorParamsAs1DForOutWhenUnconnected=off
  wires:
  data_in_i/1 -> Relational Operator/1
  Threshold Voltage/1 -> Relational Operator/2
  Disabled Input Value/1 -> Switch/3
  Switch1/1 -> data_in_o/1
  Invert/1 -> Switch1/2
  Inverter/1 -> Switch1/1
  Relational Operator/1 -> Switch/1
  Switch/1 -> Inverter/1, Switch1/3
  enable_i/1 -> Data Type Conversion/1
  Inverter1/1 -> Switch/2
  direction_i/1 -> Data Type Conversion1/1
  Inverter2/1 -> Inverter1/2
  Disabled Output Value/1 -> Switch2/3
  Inverter3/1 -> Switch2/2
  data_out_i/1 -> Switch2/1
  Invert1/1 -> Switch3/2
  Inverter4/1 -> Switch3/1
  Switch2/1 -> Inverter4/1, Switch3/3
  Switch3/1 -> Voltage/1
  Data Type Conversion/1 -> Inverter1/1, Inverter3/1
  Data Type Conversion1/1 -> Inverter2/1, Inverter3/2
  Voltage/1 -> data_out_o/1

== system SVM_test2/Subsystem/FPGA_IO_WRITE_BL18/dig_inout_tp1 ==
  note: The Digital In value is simulated by Threshold voltage detection.
  note: The nominal input range is NOT simulated because
      | the HW does not saturate according to the input range.
  data_in_i : Inport
  enable_i : Inport  Port=2
  data_out_i : Inport  Port=3
  direction_i : Inport  Port=4
  Data Type Conversion : DataTypeConversion
  Data Type Conversion1 : DataTypeConversion
  Disabled Input Value : Constant  Value=0
  Disabled Output Value : Constant  Value=0
  Invert : Constant  Value=inverted_dio
  Invert1 : Constant  Value=inverted_dio
  Inverter : Logic  Operator=NOT  AllPortsSameDT=off  OutDataTypeStr=boolean
  Inverter1 : Logic  AllPortsSameDT=off  OutDataTypeStr=boolean
  Inverter2 : Logic  Operator=NOT  AllPortsSameDT=off  OutDataTypeStr=boolean
  Inverter3 : Logic  AllPortsSameDT=off  OutDataTypeStr=boolean
  Inverter4 : Logic  Operator=NOT  AllPortsSameDT=off  OutDataTypeStr=boolean
  Relational Operator : RelationalOperator  OutDataTypeStr=boolean  RndMeth=Nearest
  Switch{,1..3} (4 alike) : Switch  Threshold=1
  Threshold Voltage : Constant  Value=2
  Voltage : Gain  Gain=voltage  ParamDataTypeStr=float('double')
  data_in_o : Outport  VectorParamsAs1DForOutWhenUnconnected=off
  data_out_o : Outport  Port=2  VectorParamsAs1DForOutWhenUnconnected=off
  wires:
  data_in_i/1 -> Relational Operator/1
  Threshold Voltage/1 -> Relational Operator/2
  Disabled Input Value/1 -> Switch/3
  Switch1/1 -> data_in_o/1
  Invert/1 -> Switch1/2
  Inverter/1 -> Switch1/1
  Relational Operator/1 -> Switch/1
  Switch/1 -> Inverter/1, Switch1/3
  enable_i/1 -> Data Type Conversion/1
  Inverter1/1 -> Switch/2
  direction_i/1 -> Data Type Conversion1/1
  Inverter2/1 -> Inverter1/2
  Disabled Output Value/1 -> Switch2/3
  Inverter3/1 -> Switch2/2
  data_out_i/1 -> Switch2/1
  Invert1/1 -> Switch3/2
  Inverter4/1 -> Switch3/1
  Switch2/1 -> Inverter4/1, Switch3/3
  Switch3/1 -> Voltage/1
  Data Type Conversion/1 -> Inverter1/1, Inverter3/1
  Data Type Conversion1/1 -> Inverter2/1, Inverter3/2
  Voltage/1 -> data_out_o/1

== system SVM_test2/Subsystem/FPGA_IO_WRITE_BL2/dig_inout_tp1 ==
  note: The Digital In value is simulated by Threshold voltage detection.
  note: The nominal input range is NOT simulated because
      | the HW does not saturate according to the input range.
  data_in_i : Inport
  enable_i : Inport  Port=2
  data_out_i : Inport  Port=3
  direction_i : Inport  Port=4
  Data Type Conversion : DataTypeConversion
  Data Type Conversion1 : DataTypeConversion
  Disabled Input Value : Constant  Value=0
  Disabled Output Value : Constant  Value=0
  Invert : Constant  Value=inverted_dio
  Invert1 : Constant  Value=inverted_dio
  Inverter : Logic  Operator=NOT  AllPortsSameDT=off  OutDataTypeStr=boolean
  Inverter1 : Logic  AllPortsSameDT=off  OutDataTypeStr=boolean
  Inverter2 : Logic  Operator=NOT  AllPortsSameDT=off  OutDataTypeStr=boolean
  Inverter3 : Logic  AllPortsSameDT=off  OutDataTypeStr=boolean
  Inverter4 : Logic  Operator=NOT  AllPortsSameDT=off  OutDataTypeStr=boolean
  Relational Operator : RelationalOperator  OutDataTypeStr=boolean  RndMeth=Nearest
  Switch{,1..3} (4 alike) : Switch  Threshold=1
  Threshold Voltage : Constant  Value=2
  Voltage : Gain  Gain=voltage  ParamDataTypeStr=float('double')
  data_in_o : Outport  VectorParamsAs1DForOutWhenUnconnected=off
  data_out_o : Outport  Port=2  VectorParamsAs1DForOutWhenUnconnected=off
  wires:
  data_in_i/1 -> Relational Operator/1
  Threshold Voltage/1 -> Relational Operator/2
  Disabled Input Value/1 -> Switch/3
  Switch1/1 -> data_in_o/1
  Invert/1 -> Switch1/2
  Inverter/1 -> Switch1/1
  Relational Operator/1 -> Switch/1
  Switch/1 -> Inverter/1, Switch1/3
  enable_i/1 -> Data Type Conversion/1
  Inverter1/1 -> Switch/2
  direction_i/1 -> Data Type Conversion1/1
  Inverter2/1 -> Inverter1/2
  Disabled Output Value/1 -> Switch2/3
  Inverter3/1 -> Switch2/2
  data_out_i/1 -> Switch2/1
  Invert1/1 -> Switch3/2
  Inverter4/1 -> Switch3/1
  Switch2/1 -> Inverter4/1, Switch3/3
  Switch3/1 -> Voltage/1
  Data Type Conversion/1 -> Inverter1/1, Inverter3/1
  Data Type Conversion1/1 -> Inverter2/1, Inverter3/2
  Voltage/1 -> data_out_o/1

== system SVM_test2/Subsystem/FPGA_IO_WRITE_BL3/dig_inout_tp1 ==
  note: The Digital In value is simulated by Threshold voltage detection.
  note: The nominal input range is NOT simulated because
      | the HW does not saturate according to the input range.
  data_in_i : Inport
  enable_i : Inport  Port=2
  data_out_i : Inport  Port=3
  direction_i : Inport  Port=4
  Data Type Conversion : DataTypeConversion
  Data Type Conversion1 : DataTypeConversion
  Disabled Input Value : Constant  Value=0
  Disabled Output Value : Constant  Value=0
  Invert : Constant  Value=inverted_dio
  Invert1 : Constant  Value=inverted_dio
  Inverter : Logic  Operator=NOT  AllPortsSameDT=off  OutDataTypeStr=boolean
  Inverter1 : Logic  AllPortsSameDT=off  OutDataTypeStr=boolean
  Inverter2 : Logic  Operator=NOT  AllPortsSameDT=off  OutDataTypeStr=boolean
  Inverter3 : Logic  AllPortsSameDT=off  OutDataTypeStr=boolean
  Inverter4 : Logic  Operator=NOT  AllPortsSameDT=off  OutDataTypeStr=boolean
  Relational Operator : RelationalOperator  OutDataTypeStr=boolean  RndMeth=Nearest
  Switch{,1..3} (4 alike) : Switch  Threshold=1
  Threshold Voltage : Constant  Value=2
  Voltage : Gain  Gain=voltage  ParamDataTypeStr=float('double')
  data_in_o : Outport  VectorParamsAs1DForOutWhenUnconnected=off
  data_out_o : Outport  Port=2  VectorParamsAs1DForOutWhenUnconnected=off
  wires:
  data_in_i/1 -> Relational Operator/1
  Threshold Voltage/1 -> Relational Operator/2
  Disabled Input Value/1 -> Switch/3
  Switch1/1 -> data_in_o/1
  Invert/1 -> Switch1/2
  Inverter/1 -> Switch1/1
  Relational Operator/1 -> Switch/1
  Switch/1 -> Inverter/1, Switch1/3
  enable_i/1 -> Data Type Conversion/1
  Inverter1/1 -> Switch/2
  direction_i/1 -> Data Type Conversion1/1
  Inverter2/1 -> Inverter1/2
  Disabled Output Value/1 -> Switch2/3
  Inverter3/1 -> Switch2/2
  data_out_i/1 -> Switch2/1
  Invert1/1 -> Switch3/2
  Inverter4/1 -> Switch3/1
  Switch2/1 -> Inverter4/1, Switch3/3
  Switch3/1 -> Voltage/1
  Data Type Conversion/1 -> Inverter1/1, Inverter3/1
  Data Type Conversion1/1 -> Inverter2/1, Inverter3/2
  Voltage/1 -> data_out_o/1

== system SVM_test2/Subsystem/FPGA_IO_WRITE_BL4/dig_inout_tp1 ==
  note: The Digital In value is simulated by Threshold voltage detection.
  note: The nominal input range is NOT simulated because
      | the HW does not saturate according to the input range.
  data_in_i : Inport
  enable_i : Inport  Port=2
  data_out_i : Inport  Port=3
  direction_i : Inport  Port=4
  Data Type Conversion : DataTypeConversion
  Data Type Conversion1 : DataTypeConversion
  Disabled Input Value : Constant  Value=0
  Disabled Output Value : Constant  Value=0
  Invert : Constant  Value=inverted_dio
  Invert1 : Constant  Value=inverted_dio
  Inverter : Logic  Operator=NOT  AllPortsSameDT=off  OutDataTypeStr=boolean
  Inverter1 : Logic  AllPortsSameDT=off  OutDataTypeStr=boolean
  Inverter2 : Logic  Operator=NOT  AllPortsSameDT=off  OutDataTypeStr=boolean
  Inverter3 : Logic  AllPortsSameDT=off  OutDataTypeStr=boolean
  Inverter4 : Logic  Operator=NOT  AllPortsSameDT=off  OutDataTypeStr=boolean
  Relational Operator : RelationalOperator  OutDataTypeStr=boolean  RndMeth=Nearest
  Switch{,1..3} (4 alike) : Switch  Threshold=1
  Threshold Voltage : Constant  Value=2
  Voltage : Gain  Gain=voltage  ParamDataTypeStr=float('double')
  data_in_o : Outport  VectorParamsAs1DForOutWhenUnconnected=off
  data_out_o : Outport  Port=2  VectorParamsAs1DForOutWhenUnconnected=off
  wires:
  data_in_i/1 -> Relational Operator/1
  Threshold Voltage/1 -> Relational Operator/2
  Disabled Input Value/1 -> Switch/3
  Switch1/1 -> data_in_o/1
  Invert/1 -> Switch1/2
  Inverter/1 -> Switch1/1
  Relational Operator/1 -> Switch/1
  Switch/1 -> Inverter/1, Switch1/3
  enable_i/1 -> Data Type Conversion/1
  Inverter1/1 -> Switch/2
  direction_i/1 -> Data Type Conversion1/1
  Inverter2/1 -> Inverter1/2
  Disabled Output Value/1 -> Switch2/3
  Inverter3/1 -> Switch2/2
  data_out_i/1 -> Switch2/1
  Invert1/1 -> Switch3/2
  Inverter4/1 -> Switch3/1
  Switch2/1 -> Inverter4/1, Switch3/3
  Switch3/1 -> Voltage/1
  Data Type Conversion/1 -> Inverter1/1, Inverter3/1
  Data Type Conversion1/1 -> Inverter2/1, Inverter3/2
  Voltage/1 -> data_out_o/1

== system SVM_test2/Subsystem/FPGA_IO_WRITE_BL5/dig_inout_tp1 ==
  note: The Digital In value is simulated by Threshold voltage detection.
  note: The nominal input range is NOT simulated because
      | the HW does not saturate according to the input range.
  data_in_i : Inport
  enable_i : Inport  Port=2
  data_out_i : Inport  Port=3
  direction_i : Inport  Port=4
  Data Type Conversion : DataTypeConversion
  Data Type Conversion1 : DataTypeConversion
  Disabled Input Value : Constant  Value=0
  Disabled Output Value : Constant  Value=0
  Invert : Constant  Value=inverted_dio
  Invert1 : Constant  Value=inverted_dio
  Inverter : Logic  Operator=NOT  AllPortsSameDT=off  OutDataTypeStr=boolean
  Inverter1 : Logic  AllPortsSameDT=off  OutDataTypeStr=boolean
  Inverter2 : Logic  Operator=NOT  AllPortsSameDT=off  OutDataTypeStr=boolean
  Inverter3 : Logic  AllPortsSameDT=off  OutDataTypeStr=boolean
  Inverter4 : Logic  Operator=NOT  AllPortsSameDT=off  OutDataTypeStr=boolean
  Relational Operator : RelationalOperator  OutDataTypeStr=boolean  RndMeth=Nearest
  Switch{,1..3} (4 alike) : Switch  Threshold=1
  Threshold Voltage : Constant  Value=2
  Voltage : Gain  Gain=voltage  ParamDataTypeStr=float('double')
  data_in_o : Outport  VectorParamsAs1DForOutWhenUnconnected=off
  data_out_o : Outport  Port=2  VectorParamsAs1DForOutWhenUnconnected=off
  wires:
  data_in_i/1 -> Relational Operator/1
  Threshold Voltage/1 -> Relational Operator/2
  Disabled Input Value/1 -> Switch/3
  Switch1/1 -> data_in_o/1
  Invert/1 -> Switch1/2
  Inverter/1 -> Switch1/1
  Relational Operator/1 -> Switch/1
  Switch/1 -> Inverter/1, Switch1/3
  enable_i/1 -> Data Type Conversion/1
  Inverter1/1 -> Switch/2
  direction_i/1 -> Data Type Conversion1/1
  Inverter2/1 -> Inverter1/2
  Disabled Output Value/1 -> Switch2/3
  Inverter3/1 -> Switch2/2
  data_out_i/1 -> Switch2/1
  Invert1/1 -> Switch3/2
  Inverter4/1 -> Switch3/1
  Switch2/1 -> Inverter4/1, Switch3/3
  Switch3/1 -> Voltage/1
  Data Type Conversion/1 -> Inverter1/1, Inverter3/1
  Data Type Conversion1/1 -> Inverter2/1, Inverter3/2
  Voltage/1 -> data_out_o/1
